simulink model "Fianl_Q4"  (R2020a)
settings: Solver=VariableStepAuto  StartTime=0.0  StopTime=10.0  RelTol=1e-3
settings Model: Creator=Joey Baby  LastModifiedBy=Joey Baby

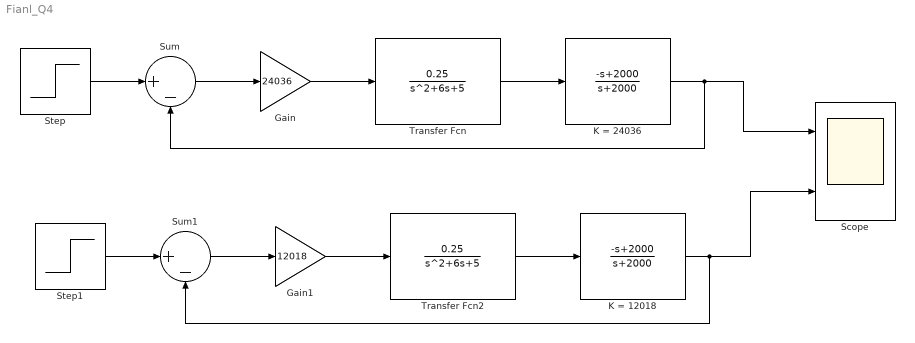
== system Fianl_Q4 ==
  Gain : Gain  Gain=24036
  Gain1 : Gain  Gain=12018
  K = 12018 : TransferFcn  Numerator=[-1 2000]  Denominator=[1 2000]
  K = 24036 : TransferFcn  Numerator=[-1 2000]  Denominator=[1 2000]
  Scope : Scope  NumInputPorts=2
  Step : Step  SampleTime=0
  Step1 : Step  SampleTime=0
  Sum : Sum  Inputs=|+-
  Sum1 : Sum  Inputs=|+-
  Transfer Fcn : TransferFcn  Numerator=[0.25]  Denominator=[1 6 5]
  Transfer Fcn2 : TransferFcn  Numerator=[0.25]  Denominator=[1 6 5]
  wires:
  Step/1 -> Sum/1
  Sum/1 -> Gain/1
  Gain/1 -> Transfer Fcn/1
  Transfer Fcn/1 -> K = 24036/1
  Gain1/1 -> Transfer Fcn2/1
  Step1/1 -> Sum1/1
  Sum1/1 -> Gain1/1
  Transfer Fcn2/1 -> K = 12018/1
  K = 24036/1 -> Sum/2, Scope/1
  K = 12018/1 -> Scope/2, Sum1/2
